simulink library "INT_GlbDa_TrqDem"  (R2016b)
settings: Solver=VariableStepAuto  StartTime=0.0  StopTime=10.0  RelTol=1e-3
settings Model: Creator=Administrator  LastModifiedBy=Administrator

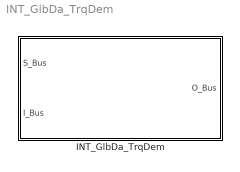
== system INT_GlbDa_TrqDem ==
  INT_GlbDa_TrqDem : Subsystem

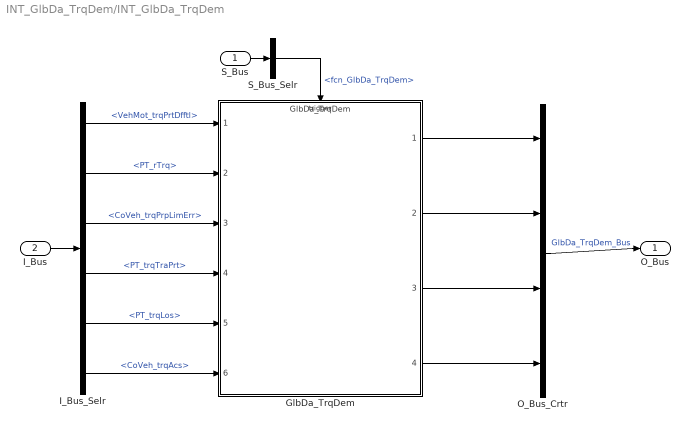
== system INT_GlbDa_TrqDem/INT_GlbDa_TrqDem ==
  S_Bus : Inport
  I_Bus : Inport  Port=2
  GlbDa_TrqDem : ModelReference  ModelNameDialog=GlbDa_TrqDem  SimulationMode=Normal  ModelReferenceVersion=1.5  TriggerPortName=function  TriggerPortTriggerType=function-call  TriggerPortStatesWhenEnabling=held
  I_Bus_Selr : BusSelector  OutputSignals=VehMot_trqPrtDfftl,PT_rTrq,CoVeh_trqPrpLimErr,PT_trqTraPrt,PT_trqLos,CoVeh_trqAcs
  O_Bus_Crtr : BusCreator  Inputs=4
  S_Bus_Selr : BusSelector  OutputSignals=fcn_GlbDa_TrqDem
  O_Bus : Outport
  wires:
  S_Bus_Selr/1 -> GlbDa_TrqDem/Trigger  "<fcn_GlbDa_TrqDem>"
  S_Bus/1 -> S_Bus_Selr/1
  I_Bus/1 -> I_Bus_Selr/1
  I_Bus_Selr/1 -> GlbDa_TrqDem/1  "<VehMot_trqPrtDfftl>"
  I_Bus_Selr/2 -> GlbDa_TrqDem/2  "<PT_rTrq>"
  I_Bus_Selr/3 -> GlbDa_TrqDem/3  "<CoVeh_trqPrpLimErr>"
  I_Bus_Selr/4 -> GlbDa_TrqDem/4  "<PT_trqTraPrt>"
  I_Bus_Selr/5 -> GlbDa_TrqDem/5  "<PT_trqLos>"
  I_Bus_Selr/6 -> GlbDa_TrqDem/6  "<CoVeh_trqAcs>"
  O_Bus_Crtr/1 -> O_Bus/1  "GlbDa_TrqDem_Bus"
  GlbDa_TrqDem/1 -> O_Bus_Crtr/1
  GlbDa_TrqDem/2 -> O_Bus_Crtr/2
  GlbDa_TrqDem/3 -> O_Bus_Crtr/3
  GlbDa_TrqDem/4 -> O_Bus_Crtr/4
